simulink model "Mixer_2"  (R2019b)
settings: Solver=VariableStepAuto  StartTime=0.0  StopTime=10.0  RelTol=1e-3
model workspace (MAT data in the model file):
  V0 = 1
settings Model: Creator=Анастасия  LastModifiedBy=Анастасия

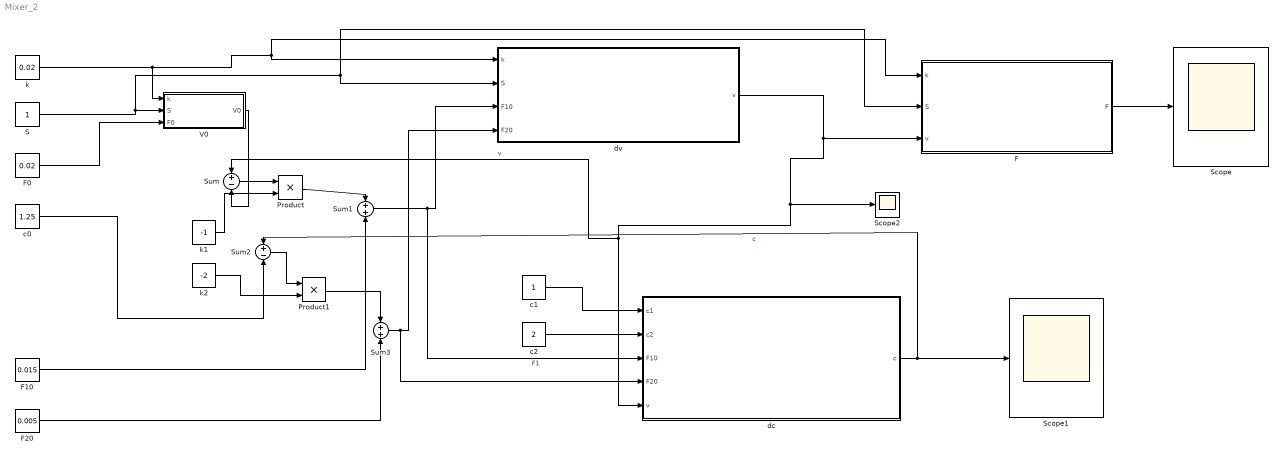
== system Mixer_2 ==
  F : Subsystem
  F0 : Constant  Value=0.02
  F10 : Constant  Value=0.015
  "F20 " : Constant  Value=0.005
  Product : Product
  Product1 : Product
  S : Constant
  Scope : Scope
  Scope1 : Scope
  Scope2 : Scope
  Sum : Sum  Inputs=+-
  Sum1 : Sum
  Sum2 : Sum  Inputs=+-
  Sum3 : Sum
  V0 : Subsystem
  "c0 " : Constant  Value=1.25
  c1 : Constant
  c2 : Constant  Value=2
  dc : Subsystem
  dv : Subsystem
  k : Constant  Value=0.02
  k1 : Constant  Value=-1
  k2 : Constant  Value=-2
  wires:
  dc/1(c) -> Sum2/1, Scope1/1  "c"
  dv/1(v) -> F/3(v), Scope2/1, Sum/1, dc/5(v)  "v"
  S/1 -> V0/2(S), F/2(S), dv/2(S)
  k/1 -> V0/1(k), F/1(k), dv/1(k)
  V0/1(V0) -> Sum/2
  F0/1 -> V0/3(F0)
  F/1(F) -> Scope/1
  Sum/1 -> Product/1
  k1/1 -> Product/2
  Product/1 -> Sum1/1
  F10/1 -> Sum1/2
  Sum1/1 -> dc/3(F10), dv/3(F10)  "F1"
  "c0 "/1 -> Sum2/2
  Sum2/1 -> Product1/1
  k2/1 -> Product1/2
  Product1/1 -> Sum3/1
  "F20 "/1 -> Sum3/2
  Sum3/1 -> dc/4(F20), dv/4(F20)
  c2/1 -> dc/2(c2)
  c1/1 -> dc/1(c1)

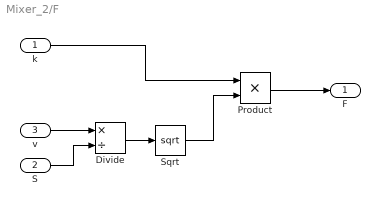
== system Mixer_2/F ==
  k : Inport
  S : Inport  Port=2
  v : Inport  Port=3
  Divide : Product  Inputs=*/
  Product : Product
  Sqrt : Sqrt  SaturateOnIntegerOverflow=on
  F : Outport
  wires:
  k/1 -> Product/1
  S/1 -> Divide/2
  Divide/1 -> Sqrt/1
  Sqrt/1 -> Product/2
  v/1 -> Divide/1
  Product/1 -> F/1

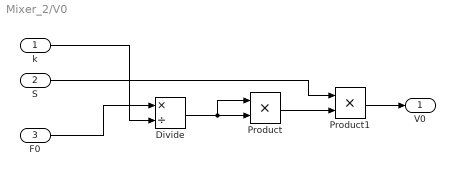
== system Mixer_2/V0 ==
  k : Inport
  S : Inport  Port=2
  F0 : Inport  Port=3
  Divide : Product  Inputs=*/
  Product : Product
  Product1 : Product
  V0 : Outport
  wires:
  F0/1 -> Divide/1
  k/1 -> Divide/2
  Divide/1 -> Product/1, Product/2
  Product/1 -> Product1/2
  S/1 -> Product1/1
  Product1/1 -> V0/1

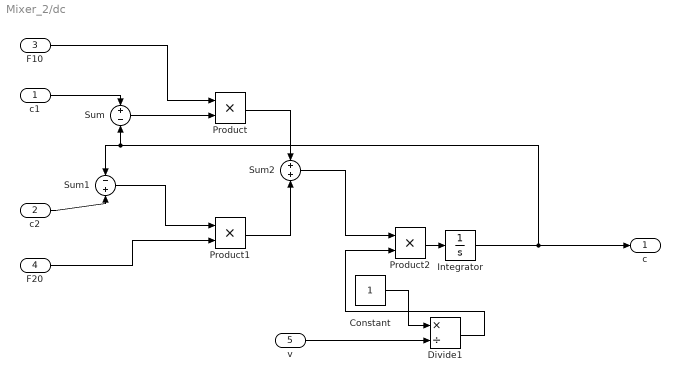
== system Mixer_2/dc ==
  c1 : Inport
  c2 : Inport  Port=2
  F10 : Inport  Port=3
  F20 : Inport  Port=4
  v : Inport  Port=5
  Constant : Constant
  Divide1 : Product  Inputs=*/
  Integrator : Integrator
  Product : Product
  Product1 : Product
  Product2 : Product
  Sum : Sum  Inputs=+-
  Sum1 : Sum  Inputs=-+
  Sum2 : Sum
  c : Outport
  wires:
  c1/1 -> Sum/1
  Integrator/1 -> Sum1/1, Sum/2, c/1
  c2/1 -> Sum1/2
  Sum/1 -> Product/2
  F10/1 -> Product/1
  Sum1/1 -> Product1/1
  F20/1 -> Product1/2
  Product/1 -> Sum2/1
  Product1/1 -> Sum2/2
  Sum2/1 -> Product2/1
  v/1 -> Divide1/2
  Product2/1 -> Integrator/1
  Constant/1 -> Divide1/1
  Divide1/1 -> Product2/2

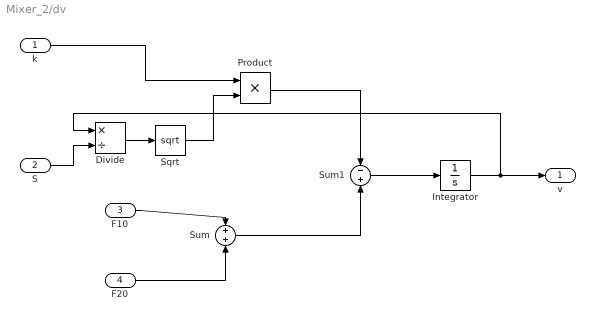
== system Mixer_2/dv ==
  k : Inport
  S : Inport  Port=2
  F10 : Inport  Port=3
  F20 : Inport  Port=4
  Divide : Product  Inputs=*/
  Integrator : Integrator  InitialCondition=1.25
  Product : Product
  Sqrt : Sqrt  SaturateOnIntegerOverflow=on
  Sum : Sum
  Sum1 : Sum  Inputs=-+
  v : Outport
  wires:
  S/1 -> Divide/2
  Divide/1 -> Sqrt/1
  Sqrt/1 -> Product/2
  k/1 -> Product/1
  F10/1 -> Sum/1
  F20/1 -> Sum/2
  Product/1 -> Sum1/1
  Sum/1 -> Sum1/2
  Sum1/1 -> Integrator/1
  Integrator/1 -> Divide/1, v/1
